simulink model "Lab_RS232b"  (Simulink 7.8)
settings: Solver=VariableStepDiscrete  StartTime=0.0  StopTime=Inf  FixedStep=Ts/4  RelTol=1e-3
PreLoadFcn:
  | clear all;
  | close all;
  | clc;
  | 
  | Txs = 1;          % Gen clk (period)
  | Trs = 1;           % Sink clk (period)
  | 
  | N = 17;    % No of characters to exchange
StartFcn:
  | clc;
  | close all;
  | 
  | TxBuffer = zeros(1,N);   % Tx characters tmp array
  | RxBuffer = ones(1,N);   % Rx characters tmp array
  | 
  | RS232_Start;
StopFcn:
  | RS232_End;
  | 
  | if size(TxBuffer) == size(RxBuffer)
  |   if TxBuffer == RxBuffer
  |     disp('OK');
  |   else
  |      disp('Error');
  |      plot(TxBuffer-RxBuffer, 'o');
  |   end
  | else
  |      disp('Error: Incorrect No of characters');
  | end
libraries: simulink x1
settings Model: Creator=theodore  LastModifiedBy=theodore
settings DebuggingCC: SolverPrmCheckMsg=none

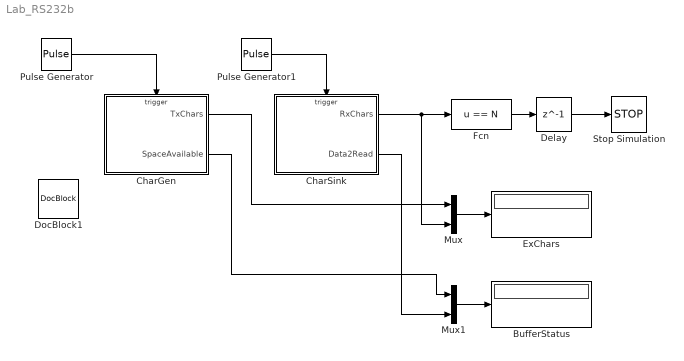
== system Lab_RS232b ==
  BufferStatus : Display
  CharGen : Stateflow chart  TreatAsAtomicUnit=on
  CharSink : Stateflow chart  TreatAsAtomicUnit=on
  Delay : Delay  DelayLength=1  SampleTime=Trs
  DocBlock1 : simulink/Model-Wide Utilities/DocBlock  DocumentType=Text
  ExChars : Display
  Fcn : Fcn  Expr=u == N
  Mux : Mux  Inputs=2
  Mux1 : Mux  Inputs=2
  Pulse Generator : DiscretePulseGenerator  PulseType=Time based  Period=Txs  PulseWidth=50  PhaseDelay=Txs/2
  Pulse Generator1 : DiscretePulseGenerator  PulseType=Time based  Period=Trs  PulseWidth=50  PhaseDelay=Trs/2
  Stop Simulation : Stop
  wires:
  Pulse Generator/1 -> CharGen/Trigger
  Pulse Generator1/1 -> CharSink/Trigger
  Fcn/1 -> Delay/1
  Mux/1 -> ExChars/1
  CharGen/1(TxChars) -> Mux/1
  CharSink/1(RxChars) -> Mux/2, Fcn/1
  Mux1/1 -> BufferStatus/1
  CharGen/2(SpaceAvailable) -> Mux1/1
  CharSink/2(Data2Read) -> Mux1/2
  Delay/1 -> Stop Simulation/1

== stateflow chart CharGen ==
  state GenState
    en: lv++;
    Val = ml.uint8(ml.rand(1)*255);
    ml.TxBuffer[lv] = Val;
    ml.d2o_s1 = Val;
    ml('DOut_1');
    TxChars = lv;
  state IniState
    en: lv = 0;
  state NoAct
  (default) -> IniState
  (junction 6) -> GenState : [ml.b2o_s1 == 0]
  (junction 7) -> GenState : [ml.b2o_s1 == 0]
  GenState -> NoAct [order 1] : [lv == ml.N]
  IniState -> (junction 6) : {ml('B2O_1'); SpaceAvailable = 1-ml.b2o_s1;}
  GenState -> (junction 7) [order 2] : [lv < ml.N]{ml('B2O_1'); SpaceAvailable = 1-ml.b2o_s1;}
  data: Val local uint8 size=1; lv local double; TxChars output double; SpaceAvailable output double
  events: TimeSlot input RISING_EDGE_EVENT

== stateflow chart CharSink ==
  state SinkState
    en: ml('DIn_2');
    Val = ml.d2r_s2;
    lv++;
    ml.RxBuffer[lv] = Val;
    RxChars = lv;
  state IniState
    en: lv = 0;
  state Idle
  (default) -> IniState
  (junction 25) -> SinkState : [ml.b2r_s2>0]
  (junction 24) -> SinkState [order 1] : [ml.b2r_s2>0]
  SinkState -> (junction 24) : {ml('B2R_2'); Data2Read = ml.b2r_s2;}
  IniState -> (junction 25) : { ml('B2R_2'); Data2Read = ml.b2r_s2;}
  (junction 24) -> Idle [order 2] : [RxChars == ml.N]{ml('B2R_2'); Data2Read = ml.b2r_s2;}
  data: Val local uint8 size=1; lv local double; RxChars output double; Data2Read output double
  events: TimeSlot input RISING_EDGE_EVENT
